simulink model "Capas"  (Simulink 6.5)
settings: Solver=ode23t  StartTime=0.0  StopTime=1  RelTol=1e-6
libraries: powerlib x1
settings Model: Creator=RS  LastModifiedBy=RS
settings SolverCC: SolverResetMethod=Robust

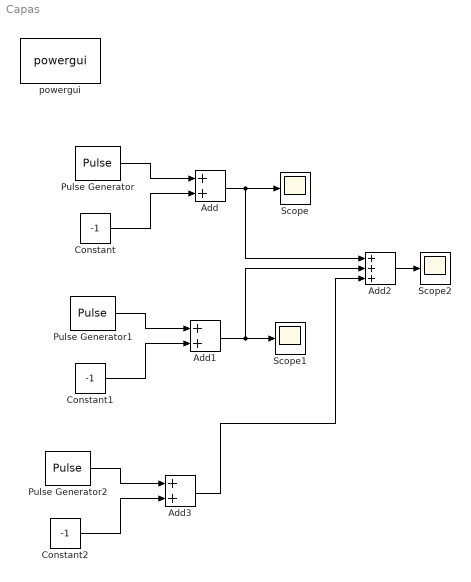
== system Capas ==
  Add : Sum  OutScaling=2^-10
  Add1 : Sum  OutScaling=2^-10
  Add2 : Sum  Inputs=+++  OutScaling=2^-10  SampleTime=10e-6
  Add3 : Sum  OutScaling=2^-10
  Constant : Constant  Value=-1  OutDataType=sfix(16)  ConRadixGroup=Use specified scaling  OutScaling=2^0  SampleTime=inf  FramePeriod=inf
  Constant1 : Constant  Value=-1  OutDataType=sfix(16)  ConRadixGroup=Use specified scaling  OutScaling=2^0  SampleTime=inf  FramePeriod=inf
  Constant2 : Constant  Value=-1  OutDataType=sfix(16)  ConRadixGroup=Use specified scaling  OutScaling=2^0  SampleTime=inf  FramePeriod=inf
  Pulse Generator : DiscretePulseGenerator  PulseType=Time based  Amplitude=2  Period=0.02  PulseWidth=50
  Pulse Generator1 : DiscretePulseGenerator  PulseType=Time based  Amplitude=2  Period=0.02  PulseWidth=50  PhaseDelay=0.02/3
  Pulse Generator2 : DiscretePulseGenerator  PulseType=Time based  Amplitude=2  Period=0.02  PulseWidth=50  PhaseDelay=0.04/3
  Scope : Scope
      settings: MaxDataPoints=10000000  SampleInput=on  SampleTime=10e-6
  Scope1 : Scope
      settings: MaxDataPoints=10000000  SampleInput=on  SampleTime=10e-6
  Scope2 : Scope
      settings: SaveName=ScopeData2  MaxDataPoints=10000000  SampleInput=on  SampleTime=10e-6
  powergui : powerlib/powergui  SystemSampleTime=-1  SimulationMode=Continuous  SampleTime=50e-6  echomessages=off  RestoreLinks=warning  x0status=blocks  Frange=[0:2:500]  Ylog=off  Xlog=on  ShowGrid=off  save=off  variable=ZData  structure=ScopeData2  ZoomFFT=off  StartTime=0.0  cycles=10  DisplayStyle=3  fundamental=50  FreqAxis=off  MaxFrequency=1000  frequencyindice=60  frequencyindicesteady=1  RmsSteady=1  display=off  Ts=0  frequency=60  methode=off  HookPort=off  Interpol=off
  wires:
  Pulse Generator/1 -> Add/1
  Constant/1 -> Add/2
  Add/1 -> Scope/1, Add2/1
  Pulse Generator1/1 -> Add1/1
  Constant1/1 -> Add1/2
  Add1/1 -> Scope1/1, Add2/2
  Add2/1 -> Scope2/1
  Pulse Generator2/1 -> Add3/1
  Constant2/1 -> Add3/2
  Add3/1 -> Add2/3
